simulink model "nms_3Dmodel_forward"  (R2017b)
settings: Solver=VariableStepAuto  StartTime=0.0  StopTime=t_end  FixedStep=1e-4  MinStep=1e-9  RelTol=1e-2  AbsTol=1e-3  EnableMultiTasking=on
InitFcn:
  | runScripts;
values from neighbouring files (symbols this model uses):
  ankle_height = 0.08    [nms_MechInit.m]
  ankleIMP = param(91+length(paramIC_opt):93+length(paramIC_opt))    [runScripts.m]
  c = 0.05    [IID_nms_MechInit.m]    (also in nms_MechInit.m)
  c_jointstop = 0.3 / (pi/180)    (= 17.1887338539)    [IID_nms_MechInit.m]    (also in nms_MechInit.m)
  CPG_On = 0    [setCPGPar.m]    (also in setCPGPar_inv.m = 1)
  CtrlPar_FP = [alpha0 alpha_cd alpha_cv]    [setCtrlPar.m]
  CtrlPar_FP_R = [R_hipR0 R_hipR_cd R_hipR_cv]    [setCtrlPar.m]
  CtrlPar_LL = l_clr    [setCtrlPar.m]
  CtrlPar_Side = [beta_cd  beta_cv]    [setCtrlPar.m]
  CtrlPar_St = [StPreStim St_M1 St_M2 St_M3 St_M4 St_M5 St_M11]    [setCtrlPar.m]
  CtrlPar_St_R = [R_StPreStim R_St_M1 R_St_M3 R_St_M4]    [setCtrlPar.m]
  CtrlPar_Sw = [SwPreStim SwPhasePari SwPhaseParii SwCtrlPar_H SwCtrlPar_A      SwCtrlPar_Ki SwCtrlPar_Kii SwCtrlPar_Kiii SwCtrlPar_StP]    [setCtrlPar.m]
  CtrlPar_Sw_R = [R_SwPreStim R_Sw_M6]    [setCtrlPar.m]
  CtrlPar_theta0 = parBlCtrl(1)      *1*pi/180    [setCtrlPar.m]
  CtrlPar_Tr = [Tr_St_sup Tr_Sw]    [setCtrlPar.m]
  CtrlPar_Tr_R = [R_Tr_St_sup R_Tr_Sw]    [setCtrlPar.m]
  D12_F = 0.16    [IID_nms_MechInit.m]    (also in nms_MechInit.m)
  D12_S = L_S    (= 0.5)    [IID_nms_MechInit.m]    (also in nms_MechInit.m = 0.46)
  D12_T = L_T    (= 0.5)    [IID_nms_MechInit.m]    (also in nms_MechInit.m = 0.46)
  D12z_T = 0.1* scalorFactor    (= 0.1)    [nms_MechInit.m]
  D13_F = 0.20    (= 0.2)    [IID_nms_MechInit.m]    (also in nms_MechInit.m)
  D1G_F = 0.14    [IID_nms_MechInit.m]    (also in nms_MechInit.m)
  D1G_HAT = 0.35    [IID_nms_MechInit.m]    (also in nms_MechInit.m)
  D1G_S = 0.3    [IID_nms_MechInit.m]    (also in nms_MechInit.m = 0.28)
  D1G_T = 0.3    [IID_nms_MechInit.m]    (also in nms_MechInit.m = 0.28)
  D1Gy_F = ankle_height*D1G_F/D12_F    (= 0.07)    [nms_MechInit.m]
  d_fBall = 0.1    [nms_MechInit.m]
  d_fHeel = 0.05    [nms_MechInit.m]
  DeltaThRef = 5e-3    (= 0.005)    [IID_nms_MechInit.m]    (also in nms_MechInit.m)
  Dist_LM23_PH = 0    [setDistPar.m]
  Dist_LM34_PH = 0    [setDistPar.m]
  Dist_On = 1    [IID_setDistPar.m]    (also in setDistPar.m)
  Dist_PDur = 0.15    [IID_setDistPar.m]    (also in setDistPar.m)
  Dist_RM23_PH = 0    [setDistPar.m]
  Dist_RM34_PH = 0    [setDistPar.m]
  Dist_StartTime = 15    [IID_setDistPar.m]    (also in setDistPar.m)
  Dist_xyzHAT_front_PH = 0    [setDistPar.m]
  Dist_xyzHAT_sag_PH = 0    [IID_setDistPar.m]    (also in setDistPar.m)
  Dist_xyzLAnkle_PH = 0    [setDistPar.m]
  Dist_xyzRAnkle_PH = 0    [setDistPar.m]
  eref = 0.04    [IID_nms_MechInit.m]    (also in nms_MechInit.m)
  FmaxBFSH = 350    [nms_MechInit.m]
  FmaxGAS = 1500    [IID_nms_MechInit.m]    (also in nms_MechInit.m)
  FmaxGLU = 1500    [IID_nms_MechInit.m]    (also in nms_MechInit.m)
  FmaxHAB = 3000    [nms_MechInit.m]
  FmaxHAD = 4500    [nms_MechInit.m]
  FmaxHAM = 3000    [IID_nms_MechInit.m]    (also in nms_MechInit.m)
  FmaxHFL = 2000    [IID_nms_MechInit.m]    (also in nms_MechInit.m)
  FmaxRF = 1200    [nms_MechInit.m]
  FmaxSOL = 4000    [IID_nms_MechInit.m]    (also in nms_MechInit.m)
  FmaxTA = 800    [IID_nms_MechInit.m]    (also in nms_MechInit.m)
  FmaxVAS = 6000    [IID_nms_MechInit.m]    (also in nms_MechInit.m)
  In_F = 0.005    [IID_nms_MechInit.m]    (also in nms_MechInit.m)
  In_HAT = 3    [IID_nms_MechInit.m]    (also in nms_MechInit.m = 2.5)
  In_S = 0.05    [IID_nms_MechInit.m]    (also in nms_MechInit.m)
  In_T = 0.15    [IID_nms_MechInit.m]    (also in nms_MechInit.m)
  init_a_tgt = 70*pi/180    (= 1.2217304764)    [setInitPar.m]
  init_a_tgtR = 90*pi/180    (= 1.57079632679)    [setInitPar.m]
  Inx_F = 0.0007    [nms_MechInit.m]
  Inx_HAT = 1.0    (= 1)    [nms_MechInit.m]
  Inx_S = 0.003    [nms_MechInit.m]
  Inx_T = 0.03    [nms_MechInit.m]
  Iny_F = 0.005    [nms_MechInit.m]
  Iny_HAT = 4.0    (= 4)    [nms_MechInit.m]
  Iny_S = 0.05    [nms_MechInit.m]
  Iny_T = 0.15    [nms_MechInit.m]
  K = 5    [IID_nms_MechInit.m]    (also in nms_MechInit.m)
  k_gn = k_gn/2    (= 39240)    [nms_MechInit.m]
  k_gt = k_gt/2    (= 3924)    [nms_MechInit.m]
  k_pressure = m_HAT * 9.81 / DeltaThRef    (= 104967)    [IID_nms_MechInit.m]    (also in nms_MechInit.m)
  leg_l = [D12_T D12_S]    [nms_MechInit.m]
  LongDelay = 0.020    (= 0.02)    [IID_setCtrlPar.m]    (also in nms_MechInit.m = 0.01)
  LongLoopDelay = 0.030    (= 0.03)    [nms_MechInit.m]
  loptBFSH = 0.12    [nms_MechInit.m]
  loptGAS = 0.05    [IID_nms_MechInit.m]    (also in nms_MechInit.m)
  loptGLU = 0.11    [IID_nms_MechInit.m]    (also in nms_MechInit.m)
  loptHAB = 0.09    [nms_MechInit.m]
  loptHAD = 0.10    (= 0.1)    [nms_MechInit.m]
  loptHAM = 0.10    (= 0.1)    [IID_nms_MechInit.m]    (also in nms_MechInit.m)
  loptHFL = 0.11    [IID_nms_MechInit.m]    (also in nms_MechInit.m)
  loptRF = 0.08    [nms_MechInit.m]
  loptSOL = 0.04    [IID_nms_MechInit.m]    (also in nms_MechInit.m)
  loptTA = 0.06    [IID_nms_MechInit.m]    (also in nms_MechInit.m)
  loptVAS = 0.08    [IID_nms_MechInit.m]    (also in nms_MechInit.m)
  lslackBFSH = 0.10    (= 0.1)    [nms_MechInit.m]
  lslackGAS = 0.40    (= 0.4)    [IID_nms_MechInit.m]    (also in nms_MechInit.m)
  lslackGLU = 0.13    [IID_nms_MechInit.m]    (also in nms_MechInit.m)
  lslackHAB = 0.07    [nms_MechInit.m]
  lslackHAD = 0.18    [nms_MechInit.m]
  lslackHAM = 0.31    [IID_nms_MechInit.m]    (also in nms_MechInit.m)
  lslackHFL = 0.10    (= 0.1)    [IID_nms_MechInit.m]    (also in nms_MechInit.m)
  lslackRF = 0.35    [nms_MechInit.m]
  lslackSOL = 0.26    [IID_nms_MechInit.m]    (also in nms_MechInit.m)
  lslackTA = 0.24    [IID_nms_MechInit.m]    (also in nms_MechInit.m)
  lslackVAS = 0.23    [IID_nms_MechInit.m]    (also in nms_MechInit.m)
  m_F = 1.25    [IID_nms_MechInit.m]    (also in nms_MechInit.m)
  m_HAT = 53.5    [IID_nms_MechInit.m]    (also in nms_MechInit.m)
  m_S = 3.5    [IID_nms_MechInit.m]    (also in nms_MechInit.m)
  m_T = 8.5    [IID_nms_MechInit.m]    (also in nms_MechInit.m)
  m_Total = m_F*2+m_S*2+m_T*2+m_HAT    (= 80)    [IID_nms_MechInit.m]    (also in nms_MechInit.m)
  massBFSH = 2    [nms_MechInit.m]
  massGAS = 0.45    [IID_nms_MechInit.m]    (also in nms_MechInit.m)
  massGLU = 1.4    [IID_nms_MechInit.m]    (also in nms_MechInit.m)
  massHAB = 1.145    [nms_MechInit.m]
  massHAD = 1.91    [nms_MechInit.m]
  massHAM = 1.82    [IID_nms_MechInit.m]    (also in nms_MechInit.m)
  massHFL = 1.87    [IID_nms_MechInit.m]    (also in nms_MechInit.m)
  massRF = 1    [nms_MechInit.m]
  massSOL = 1.36    [IID_nms_MechInit.m]    (also in nms_MechInit.m)
  massTA = 0.29    [IID_nms_MechInit.m]    (also in nms_MechInit.m)
  massVAS = 2.91    [IID_nms_MechInit.m]    (also in nms_MechInit.m)
  MidDelay = 0.010    (= 0.01)    [IID_setCtrlPar.m]    (also in nms_MechInit.m = 0.005)
  mu_slide = 0.8    [IID_nms_MechInit.m]    (also in nms_MechInit.m)
  mu_stick = 0.9    [IID_nms_MechInit.m]    (also in nms_MechInit.m)
  N = 1.5    [IID_nms_MechInit.m]    (also in cmaes_parfor.m = size(x,1); nms_MechInit.m)
  phi12_LowLimit = 70*pi/180    (= 1.2217304764)    [IID_nms_MechInit.m]    (also in nms_MechInit.m)
  phi12_UpLimit = 130*pi/180    (= 2.26892802759)    [IID_nms_MechInit.m]    (also in nms_MechInit.m)
  phi23_UpLimit = 175*pi/180    (= 3.05432619099)    [IID_nms_MechInit.m]    (also in nms_MechInit.m)
  phi34_UpLimit = 230*pi/180    (= 4.01425727959)    [IID_nms_MechInit.m]    (also in nms_MechInit.m)
  phi34R_LowLimit = -15*pi/180    (= -0.261799387799)    [nms_MechInit.m]
  ... (+115 more)
undefined symbols (not defined in the file or in its folder): Control_type, Fs_prosthesis, magnitude, sgn
libraries: mblibv1 x104, simulink x54, simulink_extras x38, nmc x30, NMCCPG_Library x17, powerlib_meascontrol x5
(part 17 of 17)

== system nms_3Dmodel_forward/Body Mechanics Layer/LLHeelCnt1/3D Contact/Kinetic Friction Model/Vector Norm ==
  vec : Inport
  Constant1 : Constant  Value=.5
  Sqrt : Math  Operator=pow  OutputSignalType=real  SaturateOnIntegerOverflow=on
  Squares : Math  Operator=square  OutputSignalType=real  SaturateOnIntegerOverflow=on
  Sum of Elements : Sum  Inputs=+
  norm : Outport
  wires:
  Constant1/1 -> Sqrt/2
  Squares/1 -> Sum of Elements/1
  Sum of Elements/1 -> Sqrt/1
  Sqrt/1 -> norm/1
  vec/1 -> Squares/1

== system nms_3Dmodel_forward/Body Mechanics Layer/LLHeelCnt1/3D Contact/Static Friction Model/Vector Norm ==
  vec : Inport
  Constant1 : Constant  Value=.5
  Sqrt : Math  Operator=pow  OutputSignalType=real  SaturateOnIntegerOverflow=on
  Squares : Math  Operator=square  OutputSignalType=real  SaturateOnIntegerOverflow=on
  Sum of Elements : Sum  Inputs=+
  norm : Outport
  wires:
  Constant1/1 -> Sqrt/2
  Squares/1 -> Sum of Elements/1
  Sum of Elements/1 -> Sqrt/1
  Sqrt/1 -> norm/1
  vec/1 -> Squares/1

== system nms_3Dmodel_forward/Body Mechanics Layer/LLHeelCnt2/3D Contact/Kinetic Friction Model/Vector Norm ==
  vec : Inport
  Constant1 : Constant  Value=.5
  Sqrt : Math  Operator=pow  OutputSignalType=real  SaturateOnIntegerOverflow=on
  Squares : Math  Operator=square  OutputSignalType=real  SaturateOnIntegerOverflow=on
  Sum of Elements : Sum  Inputs=+
  norm : Outport
  wires:
  Constant1/1 -> Sqrt/2
  Squares/1 -> Sum of Elements/1
  Sum of Elements/1 -> Sqrt/1
  Sqrt/1 -> norm/1
  vec/1 -> Squares/1

== system nms_3Dmodel_forward/Body Mechanics Layer/LLHeelCnt2/3D Contact/Static Friction Model/Vector Norm ==
  vec : Inport
  Constant1 : Constant  Value=.5
  Sqrt : Math  Operator=pow  OutputSignalType=real  SaturateOnIntegerOverflow=on
  Squares : Math  Operator=square  OutputSignalType=real  SaturateOnIntegerOverflow=on
  Sum of Elements : Sum  Inputs=+
  norm : Outport
  wires:
  Constant1/1 -> Sqrt/2
  Squares/1 -> Sum of Elements/1
  Sum of Elements/1 -> Sqrt/1
  Sqrt/1 -> norm/1
  vec/1 -> Squares/1

== system nms_3Dmodel_forward/Body Mechanics Layer/LLHeelCnt3/3D Contact/Kinetic Friction Model/Vector Norm ==
  vec : Inport
  Constant1 : Constant  Value=.5
  Sqrt : Math  Operator=pow  OutputSignalType=real  SaturateOnIntegerOverflow=on
  Squares : Math  Operator=square  OutputSignalType=real  SaturateOnIntegerOverflow=on
  Sum of Elements : Sum  Inputs=+
  norm : Outport
  wires:
  vec/1 -> Squares/1
  Sqrt/1 -> norm/1
  Sum of Elements/1 -> Sqrt/1
  Squares/1 -> Sum of Elements/1
  Constant1/1 -> Sqrt/2

== system nms_3Dmodel_forward/Body Mechanics Layer/LLHeelCnt3/3D Contact/Static Friction Model/Vector Norm ==
  vec : Inport
  Constant1 : Constant  Value=.5
  Sqrt : Math  Operator=pow  OutputSignalType=real  SaturateOnIntegerOverflow=on
  Squares : Math  Operator=square  OutputSignalType=real  SaturateOnIntegerOverflow=on
  Sum of Elements : Sum  Inputs=+
  norm : Outport
  wires:
  vec/1 -> Squares/1
  Sqrt/1 -> norm/1
  Sum of Elements/1 -> Sqrt/1
  Squares/1 -> Sum of Elements/1
  Constant1/1 -> Sqrt/2

== system nms_3Dmodel_forward/Body Mechanics Layer/LLHeelCnt4/3D Contact/Kinetic Friction Model/Vector Norm ==
  vec : Inport
  Constant1 : Constant  Value=.5
  Sqrt : Math  Operator=pow  OutputSignalType=real  SaturateOnIntegerOverflow=on
  Squares : Math  Operator=square  OutputSignalType=real  SaturateOnIntegerOverflow=on
  Sum of Elements : Sum  Inputs=+
  norm : Outport
  wires:
  vec/1 -> Squares/1
  Sqrt/1 -> norm/1
  Sum of Elements/1 -> Sqrt/1
  Squares/1 -> Sum of Elements/1
  Constant1/1 -> Sqrt/2

== system nms_3Dmodel_forward/Body Mechanics Layer/LLHeelCnt4/3D Contact/Static Friction Model/Vector Norm ==
  vec : Inport
  Constant1 : Constant  Value=.5
  Sqrt : Math  Operator=pow  OutputSignalType=real  SaturateOnIntegerOverflow=on
  Squares : Math  Operator=square  OutputSignalType=real  SaturateOnIntegerOverflow=on
  Sum of Elements : Sum  Inputs=+
  norm : Outport
  wires:
  vec/1 -> Squares/1
  Sqrt/1 -> norm/1
  Sum of Elements/1 -> Sqrt/1
  Squares/1 -> Sum of Elements/1
  Constant1/1 -> Sqrt/2

== system nms_3Dmodel_forward/Body Mechanics Layer/LLHeelCnt5/3D Contact/Kinetic Friction Model/Vector Norm ==
  vec : Inport
  Constant1 : Constant  Value=.5
  Sqrt : Math  Operator=pow  OutputSignalType=real  SaturateOnIntegerOverflow=on
  Squares : Math  Operator=square  OutputSignalType=real  SaturateOnIntegerOverflow=on
  Sum of Elements : Sum  Inputs=+
  norm : Outport
  wires:
  Constant1/1 -> Sqrt/2
  Squares/1 -> Sum of Elements/1
  Sum of Elements/1 -> Sqrt/1
  Sqrt/1 -> norm/1
  vec/1 -> Squares/1

== system nms_3Dmodel_forward/Body Mechanics Layer/LLHeelCnt5/3D Contact/Static Friction Model/Vector Norm ==
  vec : Inport
  Constant1 : Constant  Value=.5
  Sqrt : Math  Operator=pow  OutputSignalType=real  SaturateOnIntegerOverflow=on
  Squares : Math  Operator=square  OutputSignalType=real  SaturateOnIntegerOverflow=on
  Sum of Elements : Sum  Inputs=+
  norm : Outport
  wires:
  Constant1/1 -> Sqrt/2
  Squares/1 -> Sum of Elements/1
  Sum of Elements/1 -> Sqrt/1
  Sqrt/1 -> norm/1
  vec/1 -> Squares/1

== system nms_3Dmodel_forward/Body Mechanics Layer/LLHeelCnt6/3D Contact/Kinetic Friction Model/Vector Norm ==
  vec : Inport
  Constant1 : Constant  Value=.5
  Sqrt : Math  Operator=pow  OutputSignalType=real  SaturateOnIntegerOverflow=on
  Squares : Math  Operator=square  OutputSignalType=real  SaturateOnIntegerOverflow=on
  Sum of Elements : Sum  Inputs=+
  norm : Outport
  wires:
  Constant1/1 -> Sqrt/2
  Squares/1 -> Sum of Elements/1
  Sum of Elements/1 -> Sqrt/1
  Sqrt/1 -> norm/1
  vec/1 -> Squares/1

== system nms_3Dmodel_forward/Body Mechanics Layer/LLHeelCnt6/3D Contact/Static Friction Model/Vector Norm ==
  vec : Inport
  Constant1 : Constant  Value=.5
  Sqrt : Math  Operator=pow  OutputSignalType=real  SaturateOnIntegerOverflow=on
  Squares : Math  Operator=square  OutputSignalType=real  SaturateOnIntegerOverflow=on
  Sum of Elements : Sum  Inputs=+
  norm : Outport
  wires:
  Constant1/1 -> Sqrt/2
  Squares/1 -> Sum of Elements/1
  Sum of Elements/1 -> Sqrt/1
  Sqrt/1 -> norm/1
  vec/1 -> Squares/1

== system nms_3Dmodel_forward/Body Mechanics Layer/LLHeelCnt7/3D Contact/Kinetic Friction Model/Vector Norm ==
  vec : Inport
  Constant1 : Constant  Value=.5
  Sqrt : Math  Operator=pow  OutputSignalType=real  SaturateOnIntegerOverflow=on
  Squares : Math  Operator=square  OutputSignalType=real  SaturateOnIntegerOverflow=on
  Sum of Elements : Sum  Inputs=+
  norm : Outport
  wires:
  vec/1 -> Squares/1
  Sqrt/1 -> norm/1
  Sum of Elements/1 -> Sqrt/1
  Squares/1 -> Sum of Elements/1
  Constant1/1 -> Sqrt/2

== system nms_3Dmodel_forward/Body Mechanics Layer/LLHeelCnt7/3D Contact/Static Friction Model/Vector Norm ==
  vec : Inport
  Constant1 : Constant  Value=.5
  Sqrt : Math  Operator=pow  OutputSignalType=real  SaturateOnIntegerOverflow=on
  Squares : Math  Operator=square  OutputSignalType=real  SaturateOnIntegerOverflow=on
  Sum of Elements : Sum  Inputs=+
  norm : Outport
  wires:
  vec/1 -> Squares/1
  Sqrt/1 -> norm/1
  Sum of Elements/1 -> Sqrt/1
  Squares/1 -> Sum of Elements/1
  Constant1/1 -> Sqrt/2

== system nms_3Dmodel_forward/Body Mechanics Layer/LLHeelCnt8/3D Contact/Kinetic Friction Model/Vector Norm ==
  vec : Inport
  Constant1 : Constant  Value=.5
  Sqrt : Math  Operator=pow  OutputSignalType=real  SaturateOnIntegerOverflow=on
  Squares : Math  Operator=square  OutputSignalType=real  SaturateOnIntegerOverflow=on
  Sum of Elements : Sum  Inputs=+
  norm : Outport
  wires:
  vec/1 -> Squares/1
  Sqrt/1 -> norm/1
  Sum of Elements/1 -> Sqrt/1
  Squares/1 -> Sum of Elements/1
  Constant1/1 -> Sqrt/2

== system nms_3Dmodel_forward/Body Mechanics Layer/LLHeelCnt8/3D Contact/Static Friction Model/Vector Norm ==
  vec : Inport
  Constant1 : Constant  Value=.5
  Sqrt : Math  Operator=pow  OutputSignalType=real  SaturateOnIntegerOverflow=on
  Squares : Math  Operator=square  OutputSignalType=real  SaturateOnIntegerOverflow=on
  Sum of Elements : Sum  Inputs=+
  norm : Outport
  wires:
  vec/1 -> Squares/1
  Sqrt/1 -> norm/1
  Sum of Elements/1 -> Sqrt/1
  Squares/1 -> Sum of Elements/1
  Constant1/1 -> Sqrt/2

== matlab function nms_3Dmodel_forward/Body Mechanics Layer/MATLAB Function1 ==
  settings: updateMethod=DISCRETE  sampleTime=1/Fs_prosthesis
  data: u input; y output
function y = CircularBuffer(u)
%#codegen
% Function to implement a simple N element circular buffer

% Define the internal buffer variable as persistent so
% so that it will maintain its values from one time step
% to the next.
persistent buffer 
N = 10; %buffersize

% Initialize the buffer the first time through
if isempty(buffer)
    % Initialize the buffer
    buffer = zeros(N,38);
else
    buffer(2:N, :) = buffer(1:(N-1), :);
    buffer(1, :) = u;
end

% % Initialize knee state
% if isempty(state)
%     kstate = 1;
% end
    
% Output the buffer
y = buffer;

== matlab function nms_3Dmodel_forward/Body Mechanics Layer/MATLAB Function ==
  settings: updateMethod=DISCRETE  sampleTime=1/Fs_prosthesis
  data: signal input; t output; tNMC input; state output; t_stop output; type input
function [t, state, t_stop]    = knee_controller(signal, tNMC, type)
% Input U consists of:
% 1 - time
% 2-4 - acc
% 5-7 - gyro
% 8 knee angle
% 9 knee velocity
% 10-12 knee joint reaction
% 13-15 GRF LLBallF
% 16-18 GRF LMBallF
% 19-21 GRF LLHeelF
% 22-24 GRF LMHeelF
% 25 State
% 26 Moment according to NMC
%state = u(25);


subject_w = 82;
g = 9.81;
IMP = [2.1154    0.0000    0.0000    0.0909; ...
    0.1990    0.0000    1.5000    1.1380; ...
    0.01    0.0276    0.0090    0.0048]; %k, theta_0, d,
k = [3 0 0.4 0.6];
q_0 = [0 0 60 0]*pi/180;
b = [0.25 0.05 0.05 0.09];


lim = 3*pi/180;

persistent curstate counter last_switch ncycle q_entry

if isempty(counter)
    counter = 0;
    curstate = 0;
    last_switch = 0;
    ncycle = 0;
    q_entry = 0;
end

t = 0;
GRF_v = sum(signal(1, [14 17 20 23]-1))/(subject_w*g);
q = pi-signal(1,7);
qdot = -signal(1,8);
newstate = curstate;


% State space transition rules
switch curstate
    case 0 %stance flexion
        if qdot > 0 && (counter - last_switch) > 150 && GRF_v > 0.05
            newstate = 1;
            last_switch = counter;
            q_entry = q;
        end
    case 1 %late stance
        if GRF_v < 0.05
            newstate = 2;
            last_switch = counter;
        end
    case 2 %swing flexion
        if qdot < 0 && (counter - last_switch) > 50 && GRF_v < 0.05
            newstate = 3;
            last_switch = counter;
        end
    case 3 %swing extension
        if GRF_v > 0.05
            newstate = 0;
            last_switch = counter;
            ncycle = ncycle + 1;
        end
end

% create a knee stop
if q < lim
    t_stop = min(0, 10*subject_w*(q-lim));
else
    t_stop = 0;
end

curstate = newstate;

if type == 2 % FSM impedance
    t_IMP = 0;
    switch curstate
        case 0 %stance flexion
            t_IMP = (k(curstate+1)*(q-q_entry)+b(curstate+1)*qdot)*(180/pi);
        case 1 %late stance
            k_w = min(k(curstate), ((GRF_v-1)/(1-0.05))*(k(curstate)-k(curstate+2))+k(curstate));
            t_IMP = (k_w*(q-q_0(curstate+1))+b(curstate+1)*qdot)*(180/pi);
        case 2 %swing flexion
            t_IMP = (k(curstate+1)*(q-q_0(curstate+1))+b(curstate+1)*qdot)*(180/pi);
        case 3 %swing extension
            t_IMP = (k(curstate+1)*(q-q_0(curstate+1))+b(curstate+1)*qdot)*(180/pi);
    end
    if ncycle < 1
        t = tNMC;
    else
        t = t_IMP;
    end
end

if type == 1
    t = tNMC;
end

state = curstate;
counter = counter + 1;
end

== matlab function nms_3Dmodel_forward/CPG/Etc/StanceToSwitchSignal_overal/MATLAB Function ==
  data: u1 input; y output; u2 input
function y = fcn(u1, u2)
if u1 == 1
    y = 1;
elseif u2 == 2
    y = 2;
elseif u2 == 1 
    y = 3;
elseif u1 == 2
    y = 4;
else
    y = 0; 
end
